simulink library "inp"  (R2021b)
settings: Solver=VariableStepAuto  StartTime=0.0  StopTime=10.0  RelTol=1e-3
undefined symbols (not defined in the file): C_TASK_5MS_S, FALSE, KINP_AcoreReadyToSlp_flg_ovrdflg, KINP_AcoreReadyToSlp_flg_ovrdval, KINP_AllowMovThd_OTA_enum_ovrdflg, KINP_AllowMovThd_OTA_enum_ovrdval, KINP_APSAngleTarget_Deg_ovrdflg, KINP_APSAngleTarget_Deg_ovrdval, KINP_APSDecReq_mps2_ovrdflg, KINP_APSDecReq_mps2_ovrdval, KINP_APSDecReqA_flg_ovrdflg, KINP_APSDecReqA_flg_ovrdval, KINP_APSDFLL_cm_ovrdflg, KINP_APSDFLL_cm_ovrdval, KINP_APSDFLR_cm_ovrdflg, KINP_APSDFLR_cm_ovrdval, KINP_APSDRLL_cm_ovrdflg, KINP_APSDRLL_cm_ovrdval, KINP_APSDRLR_cm_ovrdflg, KINP_APSDRLR_cm_ovrdval, KINP_APSExitCondition_enum_ovrdflg, KINP_APSExitCondition_enum_ovrdval, KINP_APSHWVer_enum_ovrdflg, KINP_APSHWVer_enum_ovrdval, KINP_APSProgressPCT_pct_ovrdflg, KINP_APSProgressPCT_pct_ovrdval, KINP_APSReq_enum_ovrdflg, KINP_APSReq_enum_ovrdval, KINP_APSRQDisplay_enum_ovrdflg, KINP_APSRQDisplay_enum_ovrdval, KINP_APSRqEPASCtrl_flg_ovrdflg, KINP_APSRqEPASCtrl_flg_ovrdval, KINP_APSShiftPosnReq_enum_ovrdval, KINP_APSShiftPosnReq_enum_ovrflg, KINP_APSSpeedCMD_kph_ovrdval, KINP_APSSpeedCMD_kph_ovrflg, KINP_APSStaSystem_enum_ovrdflg, KINP_APSStaSystem_enum_ovrdval, KINP_APSSWVer_enum_ovrdflg, KINP_APSSWVer_enum_ovrdval, KINP_APSVMCReqA_flg_ovrdval, KINP_APSVMCReqA_flg_ovrflg, KINP_APSVRqEPASCtrl_flg_ovrdflg, KINP_APSVRqEPASCtrl_flg_ovrdval, KINP_AuxBattVolmV_mV_ovrdflg, KINP_AuxBattVolmV_mV_ovrdval, KINP_CAASSta_enum_ovrdflg, KINP_CAASSta_enum_ovrdval, KINP_CAASVMCReqA_flg_ovrdval, KINP_CAASVMCReqA_flg_ovrflg, KINP_Chime_enum_ovrdflg, KINP_Chime_enum_ovrdval, KINP_ClearDTCcmd_flg_ovrdflg, KINP_ClearDTCcmd_flg_ovrdval, KINP_EvccAplusPwrUpReq_flg_ovrdflg, KINP_EvccAplusPwrUpReq_flg_ovrdval, KINP_LFID_raw_ovrdval, KINP_LFID_raw_ovrflg, KINP_LRID_raw_ovrdval, KINP_MemOffsetAccX_raw16_ovrdflg ... (+118)
libraries: FVT_lib x942, hcu_lib x1
(part 27 of 31)

== system inp/INP/CAN4/SignalCheck/ZONE_R2 ==
  BHAL_outputs : Inport
  inp_CanValid_bus : Inport  Port=2
  Terminator_{1..6} (6 alike) : Terminator
  True_VHAL_ZRAPMWinRFOpenedSta_pct : Constant  Value=TRUE  OutDataTypeStr=boolean
  True_VHAL_ZRAPMWinRROpenedSta_pct : Constant  Value=TRUE  OutDataTypeStr=boolean
  True_VHAL_ZRSEATLVentSta_enum : Constant  Value=TRUE  OutDataTypeStr=boolean
  True_VHAL_ZRSEATMLVentSta_enum : Constant  Value=TRUE  OutDataTypeStr=boolean
  True_VHAL_ZRSEATMRVentSta_enum : Constant  Value=TRUE  OutDataTypeStr=boolean
  True_VHAL_ZRSEATRVentSta_enum : Constant  Value=TRUE  OutDataTypeStr=boolean
  ZRAPMWinRFOpenedSta : FVT_lib/inp/can_signal_template  SystemSampleTime=-1  VariantActivationTime=update diagram  Latency=0  AutoFrameSizeCalculation=off
      link override defval: Value=KINP_ZRAPMWinRFOpenedSta_pct_defval
      link override ovrdflg: Value=KINP_ZRAPMWinRFOpenedSta_pct_ovrdflg
      link override ovrdval: Value=KINP_ZRAPMWinRFOpenedSta_pct_ovrdval
  ZRAPMWinRROpenedSta : FVT_lib/inp/can_signal_template  SystemSampleTime=-1  VariantActivationTime=update diagram  Latency=0  AutoFrameSizeCalculation=off
      link override defval: Value=KINP_ZRAPMWinRROpenedSta_pct_defval
      link override ovrdflg: Value=KINP_ZRAPMWinRROpenedSta_pct_ovrdflg
      link override ovrdval: Value=KINP_ZRAPMWinRROpenedSta_pct_ovrdval
  ZRSEATLVentSta : FVT_lib/inp/can_signal_template  SystemSampleTime=-1  VariantActivationTime=update diagram  Latency=0  AutoFrameSizeCalculation=off
      link override defval: Value=KINP_ZRSEATLVentSta_enum_defval
      link override ovrdflg: Value=KINP_ZRSEATLVentSta_enum_ovrdflg
      link override ovrdval: Value=KINP_ZRSEATLVentSta_enum_ovrdval
  ZRSEATMLVentSta : FVT_lib/inp/can_signal_template  SystemSampleTime=-1  VariantActivationTime=update diagram  Latency=0  AutoFrameSizeCalculation=off
      link override defval: Value=KINP_ZRSEATMLVentSta_enum_defval
      link override ovrdflg: Value=KINP_ZRSEATMLVentSta_enum_ovrdflg
      link override ovrdval: Value=KINP_ZRSEATMLVentSta_enum_ovrdval
  ZRSEATMRVentSta : FVT_lib/inp/can_signal_template  SystemSampleTime=-1  VariantActivationTime=update diagram  Latency=0  AutoFrameSizeCalculation=off
      link override defval: Value=KINP_ZRSEATMRVentSta_enum_defval
      link override ovrdflg: Value=KINP_ZRSEATMRVentSta_enum_ovrdflg
      link override ovrdval: Value=KINP_ZRSEATMRVentSta_enum_ovrdval
  ZRSEATRVentSta : FVT_lib/inp/can_signal_template  SystemSampleTime=-1  VariantActivationTime=update diagram  Latency=0  AutoFrameSizeCalculation=off
      link override defval: Value=KINP_ZRSEATRVentSta_enum_defval
      link override ovrdflg: Value=KINP_ZRSEATRVentSta_enum_ovrdflg
      link override ovrdval: Value=KINP_ZRSEATRVentSta_enum_ovrdval
  slr1_{1..6} (6 alike) : BusSelector  OutputSignals=VINP_CANMsgValidZONER2_flg
  slr_VHAL_ZRAPMWinRFOpenedSta_pct : BusSelector  OutputSignals=VHAL_ZRAPMWinRFOpenedSta_pct
  slr_VHAL_ZRAPMWinRROpenedSta_pct : BusSelector  OutputSignals=VHAL_ZRAPMWinRROpenedSta_pct
  slr_VHAL_ZRSEATLVentSta_enum : BusSelector  OutputSignals=VHAL_ZRSEATLVentSta_enum
  slr_VHAL_ZRSEATMLVentSta_enum : BusSelector  OutputSignals=VHAL_ZRSEATMLVentSta_enum
  slr_VHAL_ZRSEATMRVentSta_enum : BusSelector  OutputSignals=VHAL_ZRSEATMRVentSta_enum
  slr_VHAL_ZRSEATRVentSta_enum : BusSelector  OutputSignals=VHAL_ZRSEATRVentSta_enum
  VINP_ZRAPMWinRFOpenedSta_pct : Outport
  VINP_ZRAPMWinRROpenedSta_pct : Outport  Port=2
  VINP_ZRSEATLVentSta_enum : Outport  Port=3
  VINP_ZRSEATMLVentSta_enum : Outport  Port=4
  VINP_ZRSEATMRVentSta_enum : Outport  Port=5
  VINP_ZRSEATRVentSta_enum : Outport  Port=6
  wires:
  BHAL_outputs/1 -> [BHAL_outputs]
  inp_CanValid_bus/1 -> [inp_CanValid_bus]
  [BHAL_outputs] -> slr_VHAL_ZRAPMWinRFOpenedSta_pct/1
  slr_VHAL_ZRAPMWinRFOpenedSta_pct/1 -> ZRAPMWinRFOpenedSta/1  "<VHAL_ZRAPMWinRFOpenedSta_pct>"
  True_VHAL_ZRAPMWinRFOpenedSta_pct/1 -> ZRAPMWinRFOpenedSta/2
  [inp_CanValid_bus] -> slr1_1/1
  slr1_1/1 -> ZRAPMWinRFOpenedSta/3  "<VINP_CANMsgValidZONER2_flg>"
  ZRAPMWinRFOpenedSta/1 -> VINP_ZRAPMWinRFOpenedSta_pct/1  "VINP_ZRAPMWinRFOpenedSta_pct"
  ZRAPMWinRFOpenedSta/2 -> Terminator_1/1
  [BHAL_outputs] -> slr_VHAL_ZRAPMWinRROpenedSta_pct/1
  slr_VHAL_ZRAPMWinRROpenedSta_pct/1 -> ZRAPMWinRROpenedSta/1  "<VHAL_ZRAPMWinRROpenedSta_pct>"
  True_VHAL_ZRAPMWinRROpenedSta_pct/1 -> ZRAPMWinRROpenedSta/2
  [inp_CanValid_bus] -> slr1_2/1
  slr1_2/1 -> ZRAPMWinRROpenedSta/3  "<VINP_CANMsgValidZONER2_flg>"
  ZRAPMWinRROpenedSta/1 -> VINP_ZRAPMWinRROpenedSta_pct/1  "VINP_ZRAPMWinRROpenedSta_pct"
  ZRAPMWinRROpenedSta/2 -> Terminator_2/1
  [BHAL_outputs] -> slr_VHAL_ZRSEATLVentSta_enum/1
  slr_VHAL_ZRSEATLVentSta_enum/1 -> ZRSEATLVentSta/1  "<VHAL_ZRSEATLVentSta_enum>"
  True_VHAL_ZRSEATLVentSta_enum/1 -> ZRSEATLVentSta/2
  [inp_CanValid_bus] -> slr1_3/1
  slr1_3/1 -> ZRSEATLVentSta/3  "<VINP_CANMsgValidZONER2_flg>"
  ZRSEATLVentSta/1 -> VINP_ZRSEATLVentSta_enum/1  "VINP_ZRSEATLVentSta_enum"
  ZRSEATLVentSta/2 -> Terminator_3/1
  [BHAL_outputs] -> slr_VHAL_ZRSEATMLVentSta_enum/1
  slr_VHAL_ZRSEATMLVentSta_enum/1 -> ZRSEATMLVentSta/1  "<VHAL_ZRSEATMLVentSta_enum>"
  True_VHAL_ZRSEATMLVentSta_enum/1 -> ZRSEATMLVentSta/2
  [inp_CanValid_bus] -> slr1_4/1
  slr1_4/1 -> ZRSEATMLVentSta/3  "<VINP_CANMsgValidZONER2_flg>"
  ZRSEATMLVentSta/1 -> VINP_ZRSEATMLVentSta_enum/1  "VINP_ZRSEATMLVentSta_enum"
  ZRSEATMLVentSta/2 -> Terminator_4/1
  [BHAL_outputs] -> slr_VHAL_ZRSEATMRVentSta_enum/1
  slr_VHAL_ZRSEATMRVentSta_enum/1 -> ZRSEATMRVentSta/1  "<VHAL_ZRSEATMRVentSta_enum>"
  True_VHAL_ZRSEATMRVentSta_enum/1 -> ZRSEATMRVentSta/2
  [inp_CanValid_bus] -> slr1_5/1
  slr1_5/1 -> ZRSEATMRVentSta/3  "<VINP_CANMsgValidZONER2_flg>"
  ZRSEATMRVentSta/1 -> VINP_ZRSEATMRVentSta_enum/1  "VINP_ZRSEATMRVentSta_enum"
  ZRSEATMRVentSta/2 -> Terminator_5/1
  [BHAL_outputs] -> slr_VHAL_ZRSEATRVentSta_enum/1
  slr_VHAL_ZRSEATRVentSta_enum/1 -> ZRSEATRVentSta/1  "<VHAL_ZRSEATRVentSta_enum>"
  True_VHAL_ZRSEATRVentSta_enum/1 -> ZRSEATRVentSta/2
  [inp_CanValid_bus] -> slr1_6/1
  slr1_6/1 -> ZRSEATRVentSta/3  "<VINP_CANMsgValidZONER2_flg>"
  ZRSEATRVentSta/1 -> VINP_ZRSEATRVentSta_enum/1  "VINP_ZRSEATRVentSta_enum"
  ZRSEATRVentSta/2 -> Terminator_6/1

== system inp/INP/CAN4/SignalCheck/zGW_APTC1 ==
  BHAL_outputs : Inport
  inp_CanValid_bus : Inport  Port=2
  FrntPTCLeActHeatPwr : FVT_lib/inp/can_signal_template  SystemSampleTime=-1  VariantActivationTime=update diagram  Latency=0  AutoFrameSizeCalculation=off
      link override defval: Value=KINP_FrntPTCLeActHeatPwr_W_defval
      link override ovrdflg: Value=KINP_FrntPTCLeActHeatPwr_W_ovrdflg
      link override ovrdval: Value=KINP_FrntPTCLeActHeatPwr_W_ovrdval
  FrntPTCRearLeActHeatPwr : FVT_lib/inp/can_signal_template  SystemSampleTime=-1  VariantActivationTime=update diagram  Latency=0  AutoFrameSizeCalculation=off
      link override defval: Value=KINP_FrntPTCRearLeActHeatPwr_W_defval
      link override ovrdflg: Value=KINP_FrntPTCRearLeActHeatPwr_W_ovrdflg
      link override ovrdval: Value=KINP_FrntPTCRearLeActHeatPwr_W_ovrdval
  FrntPTCRearRiActHeatPwr : FVT_lib/inp/can_signal_template  SystemSampleTime=-1  VariantActivationTime=update diagram  Latency=0  AutoFrameSizeCalculation=off
      link override defval: Value=KINP_FrntPTCRearRiActHeatPwr_W_defval
      link override ovrdflg: Value=KINP_FrntPTCRearRiActHeatPwr_W_ovrdflg
      link override ovrdval: Value=KINP_FrntPTCRearRiActHeatPwr_W_ovrdval
  FrntPTCRiActHeatPwr : FVT_lib/inp/can_signal_template  SystemSampleTime=-1  VariantActivationTime=update diagram  Latency=0  AutoFrameSizeCalculation=off
      link override defval: Value=KINP_FrntPTCRiActHeatPwr_W_defval
      link override ovrdflg: Value=KINP_FrntPTCRiActHeatPwr_W_ovrdflg
      link override ovrdval: Value=KINP_FrntPTCRiActHeatPwr_W_ovrdval
  Terminator_{1..4} (4 alike) : Terminator
  True_VHAL_FrntPTCLeActHeatPwr_W : Constant  Value=TRUE  OutDataTypeStr=boolean
  True_VHAL_FrntPTCRearLeActHeatPwr_W : Constant  Value=TRUE  OutDataTypeStr=boolean
  True_VHAL_FrntPTCRearRiActHeatPwr_W : Constant  Value=TRUE  OutDataTypeStr=boolean
  True_VHAL_FrntPTCRiActHeatPwr_W : Constant  Value=TRUE  OutDataTypeStr=boolean
  slr1_{1..4} (4 alike) : BusSelector  OutputSignals=VINP_CANMsgValidzGWAPTC1_flg
  slr_VHAL_FrntPTCLeActHeatPwr_W : BusSelector  OutputSignals=VHAL_FrntPTCLeActHeatPwr_W
  slr_VHAL_FrntPTCRearLeActHeatPwr_W : BusSelector  OutputSignals=VHAL_FrntPTCRearLeActHeatPwr_W
  slr_VHAL_FrntPTCRearRiActHeatPwr_W : BusSelector  OutputSignals=VHAL_FrntPTCRearRiActHeatPwr_W
  slr_VHAL_FrntPTCRiActHeatPwr_W : BusSelector  OutputSignals=VHAL_FrntPTCRiActHeatPwr_W
  VINP_FrntPTCLeActHeatPwr_W : Outport
  VINP_FrntPTCRearLeActHeatPwr_W : Outport  Port=2
  VINP_FrntPTCRearRiActHeatPwr_W : Outport  Port=3
  VINP_FrntPTCRiActHeatPwr_W : Outport  Port=4
  wires:
  BHAL_outputs/1 -> [BHAL_outputs]
  inp_CanValid_bus/1 -> [inp_CanValid_bus]
  [BHAL_outputs] -> slr_VHAL_FrntPTCLeActHeatPwr_W/1
  slr_VHAL_FrntPTCLeActHeatPwr_W/1 -> FrntPTCLeActHeatPwr/1  "<VHAL_FrntPTCLeActHeatPwr_W>"
  True_VHAL_FrntPTCLeActHeatPwr_W/1 -> FrntPTCLeActHeatPwr/2
  [inp_CanValid_bus] -> slr1_1/1
  slr1_1/1 -> FrntPTCLeActHeatPwr/3  "<VINP_CANMsgValidzGWAPTC1_flg>"
  FrntPTCLeActHeatPwr/1 -> VINP_FrntPTCLeActHeatPwr_W/1  "VINP_FrntPTCLeActHeatPwr_W"
  FrntPTCLeActHeatPwr/2 -> Terminator_1/1
  [BHAL_outputs] -> slr_VHAL_FrntPTCRearLeActHeatPwr_W/1
  slr_VHAL_FrntPTCRearLeActHeatPwr_W/1 -> FrntPTCRearLeActHeatPwr/1  "<VHAL_FrntPTCRearLeActHeatPwr_W>"
  True_VHAL_FrntPTCRearLeActHeatPwr_W/1 -> FrntPTCRearLeActHeatPwr/2
  [inp_CanValid_bus] -> slr1_2/1
  slr1_2/1 -> FrntPTCRearLeActHeatPwr/3  "<VINP_CANMsgValidzGWAPTC1_flg>"
  FrntPTCRearLeActHeatPwr/1 -> VINP_FrntPTCRearLeActHeatPwr_W/1  "VINP_FrntPTCRearLeActHeatPwr_W"
  FrntPTCRearLeActHeatPwr/2 -> Terminator_2/1
  [BHAL_outputs] -> slr_VHAL_FrntPTCRearRiActHeatPwr_W/1
  slr_VHAL_FrntPTCRearRiActHeatPwr_W/1 -> FrntPTCRearRiActHeatPwr/1  "<VHAL_FrntPTCRearRiActHeatPwr_W>"
  True_VHAL_FrntPTCRearRiActHeatPwr_W/1 -> FrntPTCRearRiActHeatPwr/2
  [inp_CanValid_bus] -> slr1_3/1
  slr1_3/1 -> FrntPTCRearRiActHeatPwr/3  "<VINP_CANMsgValidzGWAPTC1_flg>"
  FrntPTCRearRiActHeatPwr/1 -> VINP_FrntPTCRearRiActHeatPwr_W/1  "VINP_FrntPTCRearRiActHeatPwr_W"
  FrntPTCRearRiActHeatPwr/2 -> Terminator_3/1
  [BHAL_outputs] -> slr_VHAL_FrntPTCRiActHeatPwr_W/1
  slr_VHAL_FrntPTCRiActHeatPwr_W/1 -> FrntPTCRiActHeatPwr/1  "<VHAL_FrntPTCRiActHeatPwr_W>"
  True_VHAL_FrntPTCRiActHeatPwr_W/1 -> FrntPTCRiActHeatPwr/2
  [inp_CanValid_bus] -> slr1_4/1
  slr1_4/1 -> FrntPTCRiActHeatPwr/3  "<VINP_CANMsgValidzGWAPTC1_flg>"
  FrntPTCRiActHeatPwr/1 -> VINP_FrntPTCRiActHeatPwr_W/1  "VINP_FrntPTCRiActHeatPwr_W"
  FrntPTCRiActHeatPwr/2 -> Terminator_4/1

== system inp/INP/CAN4/SignalCheck/zGW_CANFr1 ==
  BHAL_outputs : Inport
  inp_CanValid_bus : Inport  Port=2
  COMPActualPwr : FVT_lib/inp/can_signal_template  SystemSampleTime=-1  VariantActivationTime=update diagram  Latency=0  AutoFrameSizeCalculation=off
      link override defval: Value=KINP_COMPActualPwr_W_defval
      link override ovrdflg: Value=KINP_COMPActualPwr_W_ovrdflg
      link override ovrdval: Value=KINP_COMPActualPwr_W_ovrdval
  COMPConCur : FVT_lib/inp/can_signal_template  SystemSampleTime=-1  VariantActivationTime=update diagram  Latency=0  AutoFrameSizeCalculation=off
      link override defval: Value=KINP_COMPConCur_A_defval
      link override ovrdflg: Value=KINP_COMPConCur_A_ovrdflg
      link override ovrdval: Value=KINP_COMPConCur_A_ovrdval
  COMPConVolt : FVT_lib/inp/can_signal_template  SystemSampleTime=-1  VariantActivationTime=update diagram  Latency=0  AutoFrameSizeCalculation=off
      link override defval: Value=KINP_COMPConVolt_V_defval
      link override ovrdflg: Value=KINP_COMPConVolt_V_ovrdflg
      link override ovrdval: Value=KINP_COMPConVolt_V_ovrdval
  COMPStatorSpd : FVT_lib/inp/can_signal_template  SystemSampleTime=-1  VariantActivationTime=update diagram  Latency=0  AutoFrameSizeCalculation=off
      link override defval: Value=KINP_COMPStatorSpd_rpm_defval
      link override ovrdflg: Value=KINP_COMPStatorSpd_rpm_ovrdflg
      link override ovrdval: Value=KINP_COMPStatorSpd_rpm_ovrdval
  PTC1PowerConsumption : FVT_lib/inp/can_signal_template  SystemSampleTime=-1  VariantActivationTime=update diagram  Latency=0  AutoFrameSizeCalculation=off
      link override defval: Value=KINP_PTC1PowerConsumption_kW_defval
      link override ovrdflg: Value=KINP_PTC1PowerConsumption_kW_ovrdflg
      link override ovrdval: Value=KINP_PTC1PowerConsumption_kW_ovrdval
  PTCActuPwrHSC6 : FVT_lib/inp/can_signal_template  SystemSampleTime=-1  VariantActivationTime=update diagram  Latency=0  AutoFrameSizeCalculation=off
      link override defval: Value=KINP_PTCActuPwrHSC6_enum_defval
      link override ovrdflg: Value=KINP_PTCActuPwrHSC6_enum_ovrdflg
      link override ovrdval: Value=KINP_PTCActuPwrHSC6_enum_ovrdval
  Terminator_{1..6} (6 alike) : Terminator
  True_VHAL_COMPActualPwr_W : Constant  Value=TRUE  OutDataTypeStr=boolean
  True_VHAL_COMPConCur_A : Constant  Value=TRUE  OutDataTypeStr=boolean
  True_VHAL_COMPConVolt_V : Constant  Value=TRUE  OutDataTypeStr=boolean
  True_VHAL_COMPStatorSpd_rpm : Constant  Value=TRUE  OutDataTypeStr=boolean
  True_VHAL_PTC1PowerConsumption_kW : Constant  Value=TRUE  OutDataTypeStr=boolean
  True_VHAL_PTCActuPwrHSC6_enum : Constant  Value=TRUE  OutDataTypeStr=boolean
  slr1_{1..6} (6 alike) : BusSelector  OutputSignals=VINP_CANMsgValidzGWCANFr1_flg
  slr_VHAL_COMPActualPwr_W : BusSelector  OutputSignals=VHAL_COMPActualPwr_W
  slr_VHAL_COMPConCur_A : BusSelector  OutputSignals=VHAL_COMPConCur_A
  slr_VHAL_COMPConVolt_V : BusSelector  OutputSignals=VHAL_COMPConVolt_V
  slr_VHAL_COMPStatorSpd_rpm : BusSelector  OutputSignals=VHAL_COMPStatorSpd_rpm
  slr_VHAL_PTC1PowerConsumption_kW : BusSelector  OutputSignals=VHAL_PTC1PowerConsumption_kW
  slr_VHAL_PTCActuPwrHSC6_enum : BusSelector  OutputSignals=VHAL_PTCActuPwrHSC6_enum
  VINP_COMPActualPwr_W : Outport
  VINP_COMPConCur_A : Outport  Port=2
  VINP_COMPConVolt_V : Outport  Port=3
  VINP_COMPStatorSpd_rpm : Outport  Port=4
  VINP_PTC1PowerConsumption_kW : Outport  Port=5
  VINP_PTCActuPwrHSC6_enum : Outport  Port=6
  wires:
  BHAL_outputs/1 -> [BHAL_outputs]
  inp_CanValid_bus/1 -> [inp_CanValid_bus]
  [BHAL_outputs] -> slr_VHAL_COMPActualPwr_W/1
  slr_VHAL_COMPActualPwr_W/1 -> COMPActualPwr/1  "<VHAL_COMPActualPwr_W>"
  True_VHAL_COMPActualPwr_W/1 -> COMPActualPwr/2
  [inp_CanValid_bus] -> slr1_1/1
  slr1_1/1 -> COMPActualPwr/3  "<VINP_CANMsgValidzGWCANFr1_flg>"
  COMPActualPwr/1 -> VINP_COMPActualPwr_W/1  "VINP_COMPActualPwr_W"
  COMPActualPwr/2 -> Terminator_1/1
  [BHAL_outputs] -> slr_VHAL_COMPConCur_A/1
  slr_VHAL_COMPConCur_A/1 -> COMPConCur/1  "<VHAL_COMPConCur_A>"
  True_VHAL_COMPConCur_A/1 -> COMPConCur/2
  [inp_CanValid_bus] -> slr1_2/1
  slr1_2/1 -> COMPConCur/3  "<VINP_CANMsgValidzGWCANFr1_flg>"
  COMPConCur/1 -> VINP_COMPConCur_A/1  "VINP_COMPConCur_A"
  COMPConCur/2 -> Terminator_2/1
  [BHAL_outputs] -> slr_VHAL_COMPConVolt_V/1
  slr_VHAL_COMPConVolt_V/1 -> COMPConVolt/1  "<VHAL_COMPConVolt_V>"
  True_VHAL_COMPConVolt_V/1 -> COMPConVolt/2
  [inp_CanValid_bus] -> slr1_3/1
  slr1_3/1 -> COMPConVolt/3  "<VINP_CANMsgValidzGWCANFr1_flg>"
  COMPConVolt/1 -> VINP_COMPConVolt_V/1  "VINP_COMPConVolt_V"
  COMPConVolt/2 -> Terminator_3/1
  [BHAL_outputs] -> slr_VHAL_COMPStatorSpd_rpm/1
  slr_VHAL_COMPStatorSpd_rpm/1 -> COMPStatorSpd/1  "<VHAL_COMPStatorSpd_rpm>"
  True_VHAL_COMPStatorSpd_rpm/1 -> COMPStatorSpd/2
  [inp_CanValid_bus] -> slr1_4/1
  slr1_4/1 -> COMPStatorSpd/3  "<VINP_CANMsgValidzGWCANFr1_flg>"
  COMPStatorSpd/1 -> VINP_COMPStatorSpd_rpm/1  "VINP_COMPStatorSpd_rpm"
  COMPStatorSpd/2 -> Terminator_4/1
  [BHAL_outputs] -> slr_VHAL_PTC1PowerConsumption_kW/1
  slr_VHAL_PTC1PowerConsumption_kW/1 -> PTC1PowerConsumption/1  "<VHAL_PTC1PowerConsumption_kW>"
  True_VHAL_PTC1PowerConsumption_kW/1 -> PTC1PowerConsumption/2
  [inp_CanValid_bus] -> slr1_5/1
  slr1_5/1 -> PTC1PowerConsumption/3  "<VINP_CANMsgValidzGWCANFr1_flg>"
  PTC1PowerConsumption/1 -> VINP_PTC1PowerConsumption_kW/1  "VINP_PTC1PowerConsumption_kW"
  PTC1PowerConsumption/2 -> Terminator_5/1
  [BHAL_outputs] -> slr_VHAL_PTCActuPwrHSC6_enum/1
  slr_VHAL_PTCActuPwrHSC6_enum/1 -> PTCActuPwrHSC6/1  "<VHAL_PTCActuPwrHSC6_enum>"
  True_VHAL_PTCActuPwrHSC6_enum/1 -> PTCActuPwrHSC6/2
  [inp_CanValid_bus] -> slr1_6/1
  slr1_6/1 -> PTCActuPwrHSC6/3  "<VINP_CANMsgValidzGWCANFr1_flg>"
  PTCActuPwrHSC6/1 -> VINP_PTCActuPwrHSC6_enum/1  "VINP_PTCActuPwrHSC6_enum"
  PTCActuPwrHSC6/2 -> Terminator_6/1
